simulink model "new_tf_disturbance"  (R2020b)
settings: Solver=VariableStepAuto  StartTime=0.0  StopTime=5e4  RelTol=1e-3
undefined symbols (not defined in the file or in its folder): x0
libraries: cstblocks x1
settings Model: OrderedModelArguments=off  Creator=Jamesh  LastModifiedBy=HP

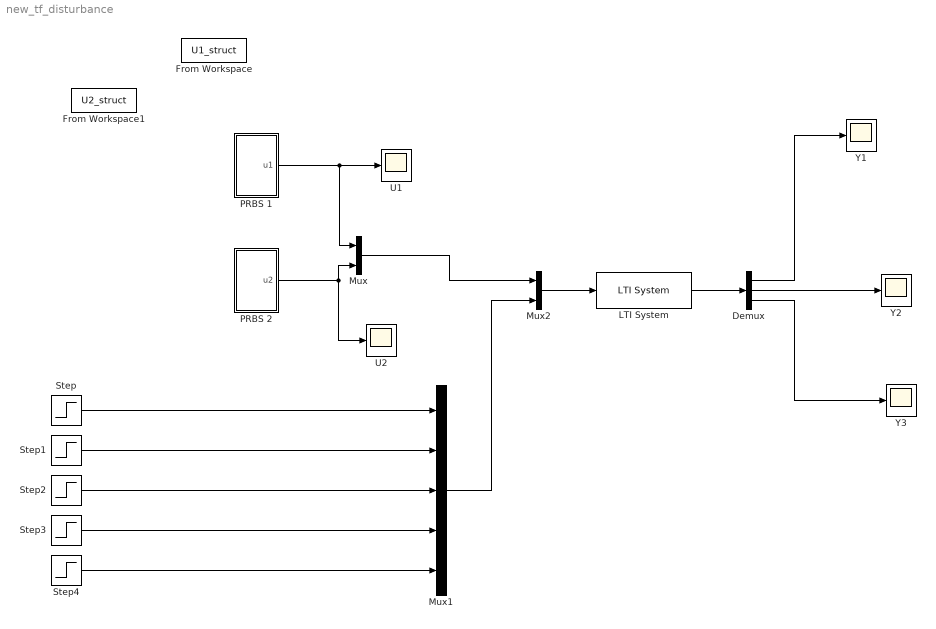
== system new_tf_disturbance ==
  Demux : Demux  Outputs=3
  From Workspace : FromWorkspace  VariableName=U1_struct
  From Workspace1 : FromWorkspace  VariableName=U2_struct
  LTI System : cstblocks/LTI System  sys=tfnew  IC=x0
  Mux : Mux  Inputs=2
  Mux1 : Mux  Inputs=5
  Mux2 : Mux  Inputs=2
  PRBS 1 : Subsystem
  PRBS 2 : Subsystem
  Step : Step  Time=0  After=x0(1)  SampleTime=0
  Step1 : Step  Time=0  After=x0(2)  SampleTime=0
  Step2 : Step  Time=0  After=x0(3)  SampleTime=0
  Step3 : Step  Time=0  After=x0(4)  SampleTime=0
  Step4 : Step  Time=0  After=x0(5)  SampleTime=0
  U1 : Scope
  U2 : Scope
  Y1 : Scope
  Y2 : Scope
  Y3 : Scope
  wires:
  LTI System/1 -> Demux/1
  Demux/1 -> Y1/1
  Demux/2 -> Y2/1
  Demux/3 -> Y3/1
  PRBS 1/1(u1) -> Mux/1, U1/1
  PRBS 2/1(u2) -> U2/1, Mux/2
  Mux/1 -> Mux2/1
  Mux1/1 -> Mux2/2
  Step/1 -> Mux1/1
  Step1/1 -> Mux1/2
  Step2/1 -> Mux1/3
  Step3/1 -> Mux1/4
  Step4/1 -> Mux1/5
  Mux2/1 -> LTI System/1

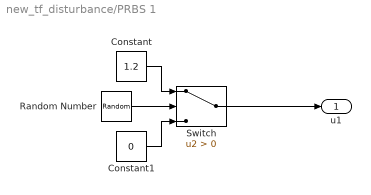
== system new_tf_disturbance/PRBS 1 ==
  Constant : Constant  Value=1.2
  Constant1 : Constant  Value=0
  Random Number : RandomNumber  Seed=1  SampleTime=0.25
  Switch : Switch  Criteria=u2 > Threshold
  u1 : Outport
  wires:
  Switch/1 -> u1/1
  Random Number/1 -> Switch/2
  Constant1/1 -> Switch/3
  Constant/1 -> Switch/1

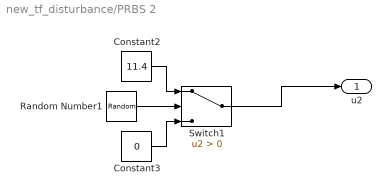
== system new_tf_disturbance/PRBS 2 ==
  Constant2 : Constant  Value=11.4
  Constant3 : Constant  Value=0
  Random Number1 : RandomNumber  Seed=2  SampleTime=0.25
  Switch1 : Switch  Criteria=u2 > Threshold
  u2 : Outport
  wires:
  Random Number1/1 -> Switch1/2
  Switch1/1 -> u2/1
  Constant3/1 -> Switch1/3
  Constant2/1 -> Switch1/1
